simulink model "controller_framework"  (R2016a)
settings: Solver=VariableStepAuto  StartTime=0.0  StopTime=10.0  RelTol=1e-3
settings Model: Creator=mikae  LastModifiedBy=mikae

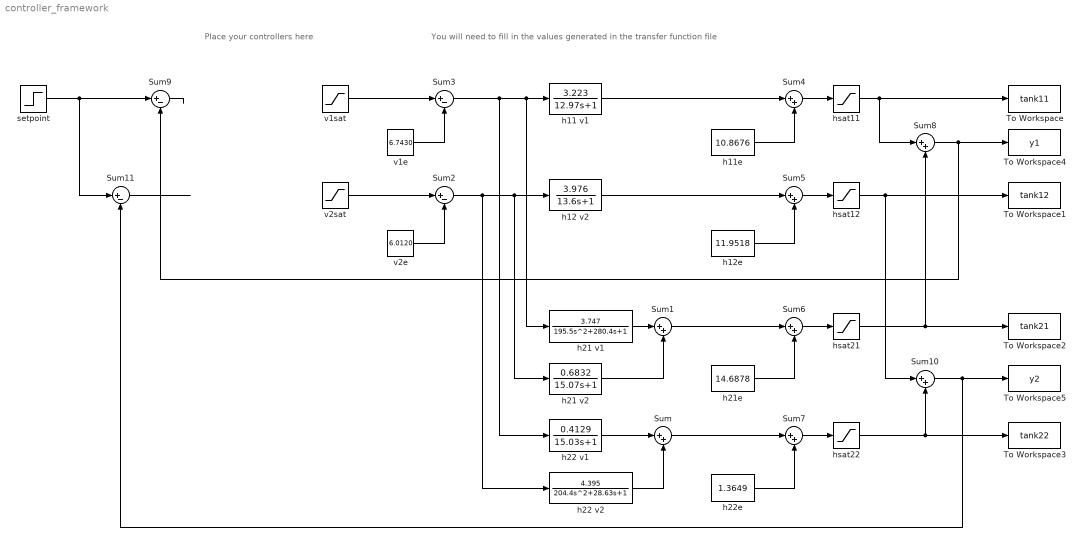
== system controller_framework ==
  note: Place your controllers here
  note: You will need to fill in the values generated in the transfer function file
  Sum{,1,4..8,10} (8 alike) : Sum  Inputs=|++
  Sum{2..3,9,11} (4 alike) : Sum  Inputs=|+-
  To Workspace : ToWorkspace  VariableName=tank11  SaveFormat=Timeseries  SampleTime=-1
  To Workspace1 : ToWorkspace  VariableName=tank12  SaveFormat=Timeseries  SampleTime=-1
  To Workspace2 : ToWorkspace  VariableName=tank21  SaveFormat=Timeseries  SampleTime=-1
  To Workspace3 : ToWorkspace  VariableName=tank22  SaveFormat=Timeseries  SampleTime=-1
  To Workspace4 : ToWorkspace  VariableName=y1  SaveFormat=Timeseries  SampleTime=-1
  To Workspace5 : ToWorkspace  VariableName=y2  SaveFormat=Timeseries  SampleTime=-1
  h11 v1 : TransferFcn  Numerator=[3.223]  Denominator=[12.97 1]
  h11e : Constant  Value=10.8676
  h12 v2 : TransferFcn  Numerator=[3.976]  Denominator=[13.6 1]
  h12e : Constant  Value=11.9518
  h21 v1 : TransferFcn  Numerator=[3.747]  Denominator=[195.5 280.4 1]
  h21 v2 : TransferFcn  Numerator=[0.6832]  Denominator=[15.07 1]
  h21e : Constant  Value=14.6878
  h22 v1 : TransferFcn  Numerator=[0.4129]  Denominator=[15.03 1]
  h22 v2 : TransferFcn  Numerator=[4.395]  Denominator=[204.4 28.63 1]
  h22e : Constant  Value=1.3649
  hsat{11..12,21..22} (4 alike) : Saturate  UpperLimit=30  LowerLimit=0
  setpoint : Step  After=26.55  SampleTime=0
  v1e : Constant  Value=6.7430
  v1sat : Saturate  UpperLimit=12  LowerLimit=0
  v2e : Constant  Value=6.0120
  v2sat : Saturate  UpperLimit=12  LowerLimit=0
  wires:
  hsat12/1 -> Sum10/1, To Workspace1/1
  hsat21/1 -> Sum8/2, To Workspace2/1
  hsat22/1 -> Sum10/2, To Workspace3/1
  ? -> v1sat/1
  ? -> v2sat/1
  h21 v1/1 -> Sum1/1
  h21 v2/1 -> Sum1/2
  h22 v1/1 -> Sum/1
  h22 v2/1 -> Sum/2
  h11 v1/1 -> Sum4/1
  Sum5/1 -> hsat12/1
  h12 v2/1 -> Sum5/1
  Sum1/1 -> Sum6/1
  Sum6/1 -> hsat21/1
  Sum/1 -> Sum7/1
  Sum7/1 -> hsat22/1
  v1sat/1 -> Sum3/1
  v2sat/1 -> Sum2/1
  Sum3/1 -> h22 v1/1, h21 v1/1, h11 v1/1
  Sum2/1 -> h22 v2/1, h21 v2/1, h12 v2/1
  h11e/1 -> Sum4/2
  h12e/1 -> Sum5/2
  h21e/1 -> Sum6/2
  h22e/1 -> Sum7/2
  v1e/1 -> Sum3/2
  v2e/1 -> Sum2/2
  hsat11/1 -> Sum8/1, To Workspace/1
  Sum4/1 -> hsat11/1
  Sum8/1 -> To Workspace4/1, Sum9/2
  Sum10/1 -> To Workspace5/1, Sum11/2
  setpoint/1 -> Sum11/1, Sum9/1
  Sum9/1 -> ?
  Sum11/1 -> ?
